simulink model "UDPKommunikation"  (R2015b)
settings: Solver=VariableStepAuto  StartTime=0.0  StopTime=inf  RelTol=1e-3
libraries: xpcrtudplib x8, xpcobsoletelib x8
settings Model: Creator=atlabor  LastModifiedBy=atlabor

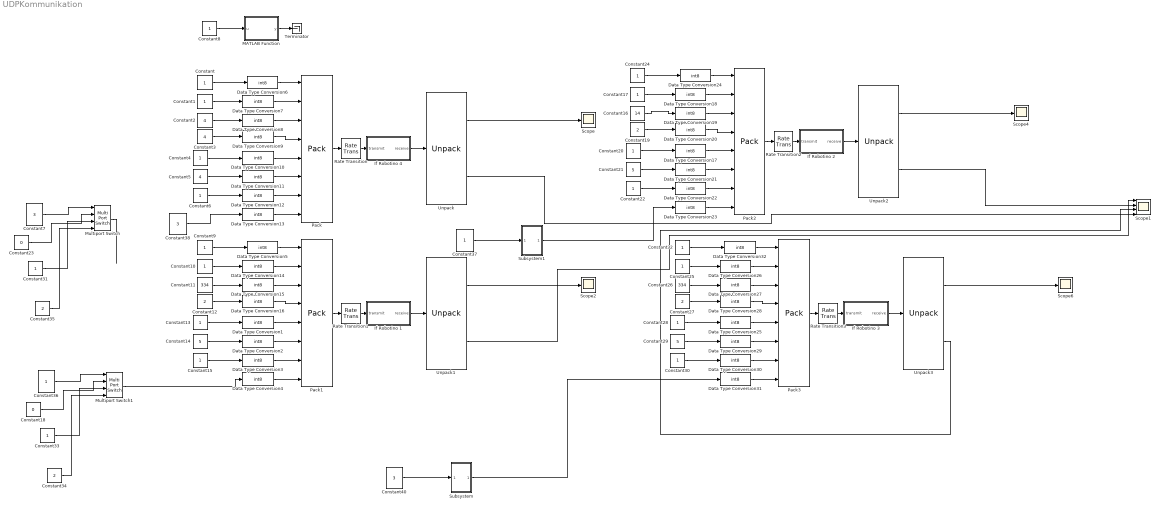
== system UDPKommunikation ==
  Constant{,1,4,6,8..10,13,15,17,20,22,24..25,28,30..33,36..37} (21 alike) : Constant
  Constant11 : Constant  Value=334
  Constant{12,19,27,34..35} (5 alike) : Constant  Value=2
  Constant14 : Constant  Value=5
  Constant16 : Constant  Value=14
  Constant18 : Constant  Value=0
  Constant2 : Constant  Value=4
  Constant21 : Constant  Value=5
  Constant23 : Constant  Value=0
  Constant26 : Constant  Value=334
  Constant29 : Constant  Value=5
  Constant3 : Constant  Value=4
  Constant38 : Constant  Value=3
  Constant40 : Constant  Value=3
  Constant5 : Constant  Value=4
  Constant7 : Constant  Value=3
  Data Type Conversion{1..32} (32 alike) : DataTypeConversion  OutDataTypeStr=int8
  If Robotino 1 : Subsystem  TreatAsAtomicUnit=on
  If Robotino 2 : Subsystem  TreatAsAtomicUnit=on
  If Robotino 3 : Subsystem  TreatAsAtomicUnit=on
  If Robotino 4 : Subsystem  TreatAsAtomicUnit=on
  MATLAB Function : MATLAB Function  TreatAsAtomicUnit=on
  Multiport Switch : MultiPortSwitch
  Multiport Switch1 : MultiPortSwitch
  Pack{,1..3} (4 alike) : xpcobsoletelib/Utilities/Pack   datatypes={'int8','int8','int8','int8','int8','int8','int8','int8'}  byteAlign=1
  Rate Transition{,1..3} (4 alike) : RateTransition  OutPortSampleTime=0.5
  Scope{,2,4,6} (4 alike) : Scope
  Scope1 : Scope  NumInputPorts=4
  Subsystem : Subsystem
  Subsystem1 : Subsystem
  Terminator : Terminator
  Unpack{,1..3} (4 alike) : xpcobsoletelib/Utilities/Unpack   dimensions={1, 1}  datatypes={'uint8','uint8'}  byteAlign=1
  wires:
  Constant/1 -> Data Type Conversion6/1
  Pack/1 -> Rate Transition/1
  Data Type Conversion6/1 -> Pack/1
  If Robotino 4/1(receive) -> Unpack/1
  Data Type Conversion7/1 -> Pack/2
  Data Type Conversion8/1 -> Pack/3
  Data Type Conversion9/1 -> Pack/4
  Data Type Conversion10/1 -> Pack/5
  Data Type Conversion11/1 -> Pack/6
  Data Type Conversion13/1 -> Pack/8
  Data Type Conversion12/1 -> Pack/7
  Constant1/1 -> Data Type Conversion7/1
  Constant3/1 -> Data Type Conversion9/1
  Constant4/1 -> Data Type Conversion10/1
  Constant5/1 -> Data Type Conversion11/1
  Constant6/1 -> Data Type Conversion12/1
  Unpack/1 -> Scope/1
  Rate Transition/1 -> If Robotino 4/1(transmit)
  Constant8/1 -> MATLAB Function/1(u)
  MATLAB Function/1(y) -> Terminator/1
  Constant9/1 -> Data Type Conversion5/1
  Pack1/1 -> Rate Transition1/1
  Data Type Conversion5/1 -> Pack1/1
  If Robotino 1/1(receive) -> Unpack1/1
  Data Type Conversion14/1 -> Pack1/2
  Data Type Conversion15/1 -> Pack1/3
  Data Type Conversion16/1 -> Pack1/4
  Data Type Conversion1/1 -> Pack1/5
  Data Type Conversion2/1 -> Pack1/6
  Data Type Conversion4/1 -> Pack1/8
  Data Type Conversion3/1 -> Pack1/7
  Constant10/1 -> Data Type Conversion14/1
  Constant11/1 -> Data Type Conversion15/1
  Constant12/1 -> Data Type Conversion16/1
  Constant13/1 -> Data Type Conversion1/1
  Constant14/1 -> Data Type Conversion2/1
  Constant15/1 -> Data Type Conversion3/1
  Unpack1/1 -> Scope2/1
  Unpack1/2 -> Scope1/1
  Rate Transition1/1 -> If Robotino 1/1(transmit)
  Constant24/1 -> Data Type Conversion24/1
  Pack2/1 -> Rate Transition2/1
  Data Type Conversion24/1 -> Pack2/1
  If Robotino 2/1(receive) -> Unpack2/1
  Data Type Conversion18/1 -> Pack2/2
  Data Type Conversion19/1 -> Pack2/3
  Data Type Conversion20/1 -> Pack2/4
  Data Type Conversion17/1 -> Pack2/5
  Data Type Conversion21/1 -> Pack2/6
  Data Type Conversion23/1 -> Pack2/8
  Data Type Conversion22/1 -> Pack2/7
  Constant17/1 -> Data Type Conversion18/1
  Constant2/1 -> Data Type Conversion8/1
  Constant19/1 -> Data Type Conversion20/1
  Constant20/1 -> Data Type Conversion17/1
  Constant21/1 -> Data Type Conversion21/1
  Constant22/1 -> Data Type Conversion22/1
  Unpack2/1 -> Scope4/1
  Unpack2/2 -> Scope1/2
  Rate Transition2/1 -> If Robotino 2/1(transmit)
  Constant32/1 -> Data Type Conversion32/1
  Pack3/1 -> Rate Transition3/1
  Data Type Conversion32/1 -> Pack3/1
  If Robotino 3/1(receive) -> Unpack3/1
  Data Type Conversion26/1 -> Pack3/2
  Data Type Conversion27/1 -> Pack3/3
  Data Type Conversion28/1 -> Pack3/4
  Data Type Conversion25/1 -> Pack3/5
  Data Type Conversion29/1 -> Pack3/6
  Data Type Conversion31/1 -> Pack3/8
  Data Type Conversion30/1 -> Pack3/7
  Constant25/1 -> Data Type Conversion26/1
  Constant26/1 -> Data Type Conversion27/1
  Constant27/1 -> Data Type Conversion28/1
  Constant28/1 -> Data Type Conversion25/1
  Constant29/1 -> Data Type Conversion29/1
  Constant30/1 -> Data Type Conversion30/1
  Unpack3/1 -> Scope6/1
  Unpack3/2 -> Scope1/3
  Rate Transition3/1 -> If Robotino 3/1(transmit)
  Constant16/1 -> Data Type Conversion19/1
  Unpack/2 -> Scope1/4
  Multiport Switch/1 -> ?
  Constant31/1 -> Multiport Switch/3
  Constant7/1 -> Multiport Switch/1
  Constant23/1 -> Multiport Switch/2
  Constant35/1 -> Multiport Switch/4
  Multiport Switch1/1 -> Data Type Conversion4/1
  Constant33/1 -> Multiport Switch1/3
  Constant36/1 -> Multiport Switch1/1
  Constant18/1 -> Multiport Switch1/2
  Constant34/1 -> Multiport Switch1/4
  Constant40/1 -> Subsystem/1(In1)
  Subsystem/1(Out1) -> Data Type Conversion31/1
  Constant37/1 -> Subsystem1/1(In1)
  Subsystem1/1(Out1) -> Data Type Conversion23/1
  Constant38/1 -> Data Type Conversion13/1

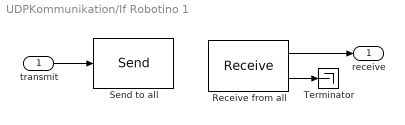
== system UDPKommunikation/If Robotino 1 ==
  transmit : Inport
  Receive from all : xpcrtudplib/Legacy UDP/Receive   ipAddress=192.168.0.11  ipPort=25010  width=2  vblLen=off  sampletime=-1
  Send to all : xpcrtudplib/Legacy UDP/Send   ipAddress=192.168.0.11  ipPort=25011  localPort=-1  vblLen=off  sampletime=-1
  Terminator : Terminator
  receive : Outport
  wires:
  Receive from all/1 -> receive/1
  Receive from all/2 -> Terminator/1
  transmit/1 -> Send to all/1

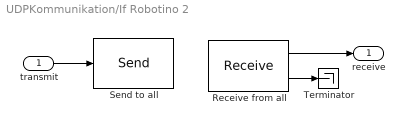
== system UDPKommunikation/If Robotino 2 ==
  transmit : Inport
  Receive from all : xpcrtudplib/Legacy UDP/Receive   ipAddress=192.168.0.12  ipPort=25020  width=2  vblLen=off  sampletime=-1
  Send to all : xpcrtudplib/Legacy UDP/Send   ipAddress=192.168.0.12  ipPort=25012  localPort=-1  vblLen=off  sampletime=-1
  Terminator : Terminator
  receive : Outport
  wires:
  transmit/1 -> Send to all/1
  Receive from all/2 -> Terminator/1
  Receive from all/1 -> receive/1

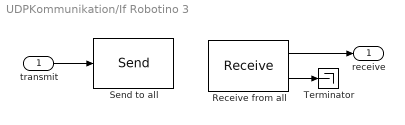
== system UDPKommunikation/If Robotino 3 ==
  transmit : Inport
  Receive from all : xpcrtudplib/Legacy UDP/Receive   ipAddress=192.168.0.13  ipPort=25030  width=2  vblLen=off  sampletime=-1
  Send to all : xpcrtudplib/Legacy UDP/Send   ipAddress=192.168.0.13  ipPort=25013  localPort=-1  vblLen=off  sampletime=-1
  Terminator : Terminator
  receive : Outport
  wires:
  transmit/1 -> Send to all/1
  Receive from all/2 -> Terminator/1
  Receive from all/1 -> receive/1

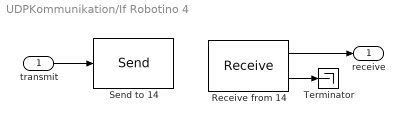
== system UDPKommunikation/If Robotino 4 ==
  transmit : Inport
  Receive from 14 : xpcrtudplib/Legacy UDP/Receive   ipAddress=192.168.0.14  ipPort=25040  width=2  vblLen=off  sampletime=-1
  Send to 14 : xpcrtudplib/Legacy UDP/Send   ipAddress=192.168.0.14  ipPort=25014  localPort=-1  vblLen=off  sampletime=-1
  Terminator : Terminator
  receive : Outport
  wires:
  transmit/1 -> Send to 14/1
  Receive from 14/2 -> Terminator/1
  Receive from 14/1 -> receive/1

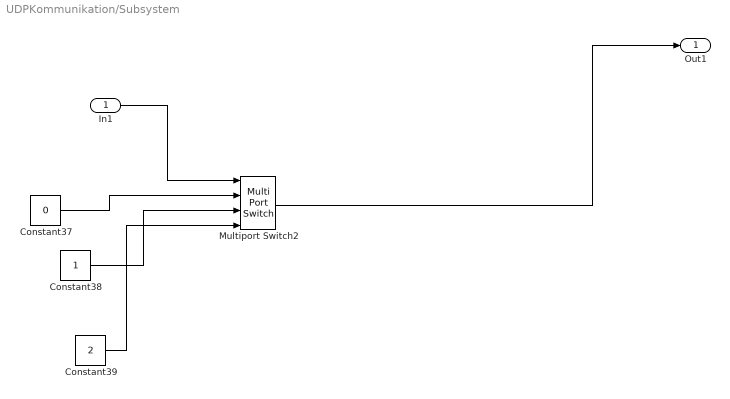
== system UDPKommunikation/Subsystem ==
  In1 : Inport
  Constant37 : Constant  Value=0
  Constant38 : Constant
  Constant39 : Constant  Value=2
  Multiport Switch2 : MultiPortSwitch
  Out1 : Outport
  wires:
  Multiport Switch2/1 -> Out1/1
  Constant37/1 -> Multiport Switch2/2
  Constant38/1 -> Multiport Switch2/3
  In1/1 -> Multiport Switch2/1
  Constant39/1 -> Multiport Switch2/4

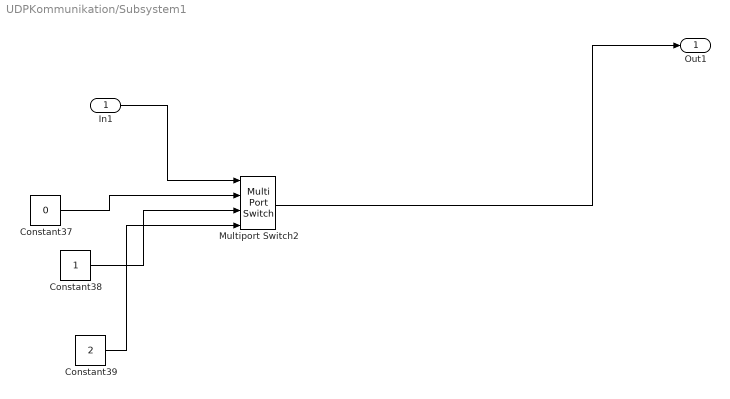
== system UDPKommunikation/Subsystem1 ==
  In1 : Inport
  Constant37 : Constant  Value=0
  Constant38 : Constant
  Constant39 : Constant  Value=2
  Multiport Switch2 : MultiPortSwitch
  Out1 : Outport
  wires:
  Constant39/1 -> Multiport Switch2/4
  In1/1 -> Multiport Switch2/1
  Constant38/1 -> Multiport Switch2/3
  Constant37/1 -> Multiport Switch2/2
  Multiport Switch2/1 -> Out1/1

== matlab function UDPKommunikation/MATLAB Function ==
  data: u input; y output
function y = fcn(u)
%#codegen
pause(1)
y = u;
